simulink model "LQG"  (R2023a)
settings: Solver=ode4  StartTime=0.0  StopTime=10  FixedStep=Ts  RelTol=1e-3
values from neighbouring files (symbols this model uses):
  K_d = dlqr(Ad, Bd, Q, R)    [controller.m]    (also in statespace.m)
  L_d = dlqe(Ad, G, Cd, wk, vk)    [controller.m]    (also in statespace.m)
  N = 1 / (Cd * inv(1 - (Ad - Bd * K_d)) * Bd)    [controller.m]    (also in tuning_wk.m = length(Z))
  Ts = 0.01    [controller.m]    (also in statespace.m)
undefined symbols (not defined in the file or in its folder): Ad, Bd, Cd, Dd
settings Model: Creator=ASUS  LastModifiedBy=Thu

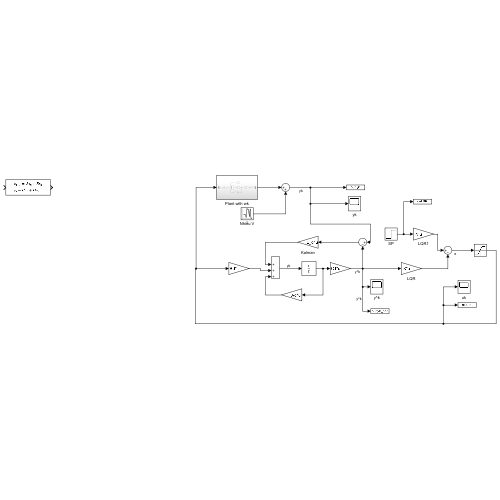
[thumbnail: Simulink's stored preview of the top-level diagram]
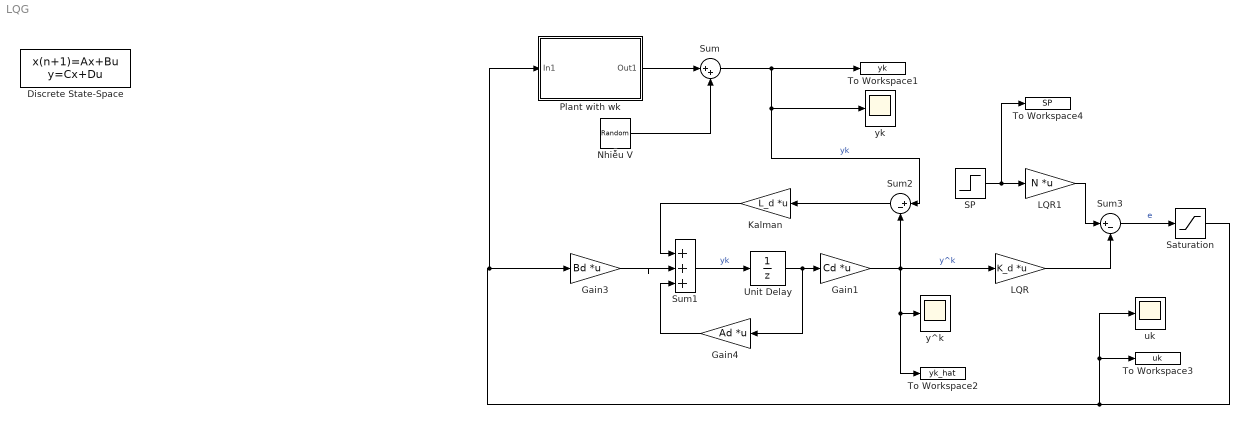
== system LQG ==
  Discrete State-Space : DiscreteStateSpace  A=Ad  B=Bd  C=Cd  D=Dd  SampleTime=0.01
  Gain1 : Gain  Gain=Cd  Multiplication=Matrix(K*u)
  Gain3 : Gain  Gain=Bd  Multiplication=Matrix(K*u)
  Gain4 : Gain  Gain=Ad  Multiplication=Matrix(K*u)
  Kalman : Gain  Gain=L_d  Multiplication=Matrix(K*u)
  LQR : Gain  Gain=K_d  Multiplication=Matrix(K*u)
  LQR1 : Gain  Gain=N  Multiplication=Matrix(K*u)
  Nhiễu V : RandomNumber  Variance=10.3505*Ts  SampleTime=Ts
  Plant with wk : Subsystem
  SP : Step  After=200  SampleTime=0.01
  Saturation : Saturate  UpperLimit=999  LowerLimit=0
  Sum : Sum  Inputs=|++
  Sum1 : Sum  Inputs=|+++
  Sum2 : Sum  Inputs=|+-
  Sum3 : Sum  Inputs=|+-
  To Workspace1 : ToWorkspace  VariableName=yk  SaveFormat=Timeseries  SampleTime=-1
  To Workspace2 : ToWorkspace  VariableName=yk_hat  SaveFormat=Timeseries  SampleTime=-1
  To Workspace3 : ToWorkspace  VariableName=uk  SaveFormat=Timeseries  SampleTime=-1
  To Workspace4 : ToWorkspace  VariableName=SP  SaveFormat=Timeseries  SampleTime=-1
  Unit Delay : UnitDelay  SampleTime=Ts  HasFrameUpgradeWarning=on
  uk : Scope
  y^k : Scope
  yk : Scope
  wires:
  Nhiễu V/1 -> Sum/2
  Sum/1 -> Sum2/1, yk/1, To Workspace1/1  "yk"
  Plant with wk/1(Out1) -> Sum/1
  Gain1/1 -> y^k/1, To Workspace2/1, LQR/1, Sum2/2  "y^k"
  Unit Delay/1 -> Gain4/1, Gain1/1
  Sum1/1 -> Unit Delay/1  "yk"
  Sum2/1 -> Kalman/1
  Kalman/1 -> Sum1/1
  Gain3/1 -> Sum1/2
  Gain4/1 -> Sum1/3
  Sum3/1 -> Saturation/1  "e"
  Saturation/1 -> To Workspace3/1, uk/1, Plant with wk/1(In1), Gain3/1
  LQR/1 -> Sum3/2
  SP/1 -> To Workspace4/1, LQR1/1
  LQR1/1 -> Sum3/1

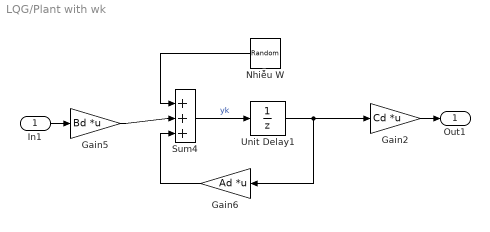
== system LQG/Plant with wk ==
  In1 : Inport
  Gain2 : Gain  Gain=Cd  Multiplication=Matrix(K*u)
  Gain5 : Gain  Gain=Bd  Multiplication=Matrix(K*u)
  Gain6 : Gain  Gain=Ad  Multiplication=Matrix(K*u)
  Nhiễu W : RandomNumber  Variance=2.0701*Ts  SampleTime=Ts
  Sum4 : Sum  Inputs=|+++
  Unit Delay1 : UnitDelay  SampleTime=Ts  HasFrameUpgradeWarning=on
  Out1 : Outport
  wires:
  Nhiễu W/1 -> Sum4/1
  Sum4/1 -> Unit Delay1/1  "yk"
  Unit Delay1/1 -> Gain2/1, Gain6/1
  Gain6/1 -> Sum4/3
  Gain5/1 -> Sum4/2
  Gain2/1 -> Out1/1
  In1/1 -> Gain5/1
